simulink model "bar"  (R2020a)
settings: Solver=ode45  StartTime=0.0  StopTime=tfinal  RelTol=1e-6  EnableMultiTasking=on
values from neighbouring files (symbols this model uses):
  Ts = mean(diff(ts))    [bar_simulation.m]
undefined symbols (not defined in the file or in its folder): Atrue, Btrue, Ctrue, Dtrue
settings Model: Creator=jomle  LastModifiedBy=franc
settings DataIOCC: LimitDataPoints=on  SaveFormat=Array  ReturnWorkspaceOutputs=off
settings OptimizationCC: LifeSpan=inf
settings DebuggingCC: SFUnexpectedBacktrackingDiag=warning  SFNoUnconditionalDefaultTransitionDiag=warning  SFExecutionAtInitializationDiag=none  ArithmeticOperatorsInVariantConditions=warning
settings HardwareCC: ProdBitPerPointer=32  ProdBitPerSizeT=32  ProdBitPerPtrDiffT=32  ProdLargestAtomicFloat=None  ProdIntDivRoundTo=Undefined  ProdEndianess=Unspecified  ProdWordSize=32  ProdHWDeviceType=32-bit Generic
settings ModelReferenceCC: PropagateSignalLabelsOutOfModel=off
settings SFSimCC: SimUseLocalCustomCode=off  CustomCodeUndefinedFunction=UseInterfaceOnly
settings RTWCC: RTWUseLocalCustomCode=off
settings CodeAppCC: StateflowObjectComments=on
settings GRTTargetCC: TargetLangStandard=C89/C90 (ANSI)
settings ConfigComp: CovMetricSettings=dw  CovHtmlReporting=on  CovSaveCumulativeToWorkspaceVar=on  CovSaveSingleToWorkspaceVar=on  CovExternalEMLEnable=off

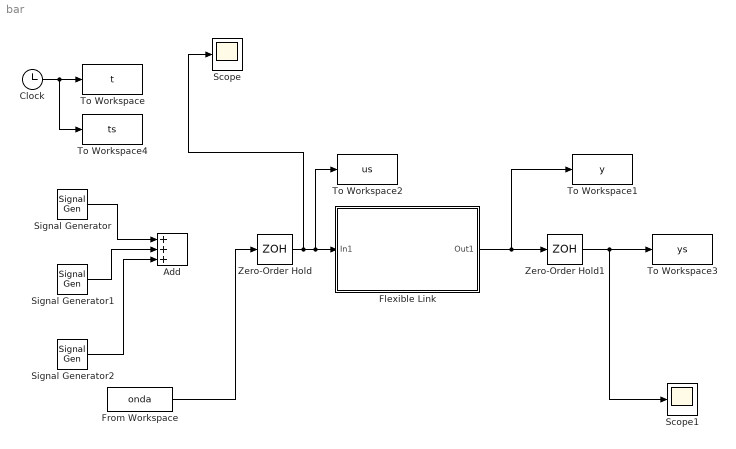
== system bar ==
  Add : Sum  Inputs=+++
  Clock : Clock
  Flexible Link : Subsystem
      mask Display: image('quanserlink.jpg')
  From Workspace : FromWorkspace  VariableName=onda
  Scope : Scope
  Scope1 : Scope
  Signal Generator : SignalGenerator  WaveForm=square  Units=rad/sec
  Signal Generator1 : SignalGenerator  WaveForm=square  Amplitude=0.2  Frequency=10  Units=rad/sec
  Signal Generator2 : SignalGenerator  WaveForm=square  Amplitude=0.2  Frequency=50  Units=rad/sec
  To Workspace : ToWorkspace  VariableName=t  SampleTime=-1
  To Workspace1 : ToWorkspace  VariableName=y  SampleTime=-1
  To Workspace2 : ToWorkspace  VariableName=us  SampleTime=Ts
  To Workspace3 : ToWorkspace  VariableName=ys  SampleTime=Ts
  To Workspace4 : ToWorkspace  VariableName=ts  SampleTime=Ts
  Zero-Order Hold : ZeroOrderHold  SampleTime=Ts
  Zero-Order Hold1 : ZeroOrderHold  SampleTime=Ts
  wires:
  Clock/1 -> To Workspace4/1, To Workspace/1
  Flexible Link/1(Out1) -> Zero-Order Hold1/1, To Workspace1/1
  Zero-Order Hold/1 -> Scope/1, To Workspace2/1, Flexible Link/1(In1)
  Signal Generator/1 -> Add/1
  Signal Generator1/1 -> Add/2
  Signal Generator2/1 -> Add/3
  From Workspace/1 -> Zero-Order Hold/1
  Zero-Order Hold1/1 -> Scope1/1, To Workspace3/1

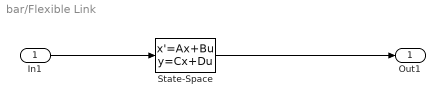
== system bar/Flexible Link ==
  In1 : Inport
  State-Space : StateSpace  A=Atrue  B=Btrue  C=Ctrue  D=Dtrue  InitialCondition=0
  Out1 : Outport
  wires:
  State-Space/1 -> Out1/1
  In1/1 -> State-Space/1
